simulink model "plataforma"  (R2015a)
settings: Solver=ode45  StartTime=0.0  StopTime=tf  MaxStep=1e-1  RelTol=1e-3
InitFcn:
  | c = clock;
  | seed_offset = c(6);
  | seed_offset = floor(seed_offset);
values from neighbouring files (symbols this model uses):
  Ts = 0.05    [Estimador.m]    (also in Estimador2.m; gerar_realizacao.m; ler_realizacao.m)
settings Model: Creator=marcos  LastModifiedBy=marcos

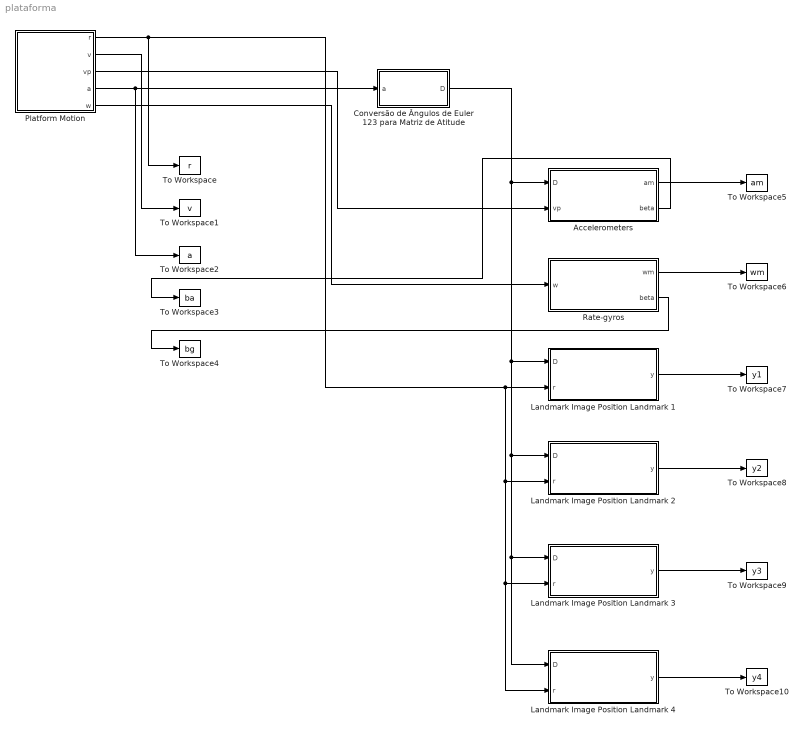
== system plataforma ==
  Accelerometers : Subsystem  mask{beta=zeros(3,1), sigma=0.0039, seed=1+seed_offset}
      mask prompts: beta "Bias (beta)"; sigma "Noise std. dev. (sigma)"
  Conversão de Ângulos de Euler 123 para Matriz de Atitude : MATLAB Function  TreatAsAtomicUnit=on
  Landmark Image Position Landmark 1 : Subsystem  mask{f=1, Dcp=[1 0 0;0 -1 0;0 0 -1], rcp_P=[0 0 0]', sigma=6e-3, p=[0 0 0]', seed=3+seed_offset}
      mask prompts: f "Comprimento focal (f)"; Dcp "Orientação da câmera (Dcp)"; rcp_P "Posição da câmera (rcp)"; sigma "Dev. padrão do ruído (sigma)"; p "Posição da landmark (p)"
  Landmark Image Position Landmark 2 : Subsystem  mask{f=1, Dcp=[1 0 0;0 -1 0;0 0 -1], rcp_P=[0 0 0]', sigma=6e-3, p=[5 5 0]', seed=4+seed_offset}
      mask prompts: f "Comprimento focal (f)"; Dcp "Orientação da câmera (Dcp)"; rcp_P "Posição da câmera (rcp)"; sigma "Dev. padrão do ruído (sigma)"; p "Posição da landmark (p)"
  Landmark Image Position Landmark 3 : Subsystem  mask{f=1, Dcp=[1 0 0;0 -1 0;0 0 -1], rcp_P=[0 0 0]', sigma=6e-3, p=[-5 5 0]', seed=5+seed_offset}
      mask prompts: f "Comprimento focal (f)"; Dcp "Orientação da câmera (Dcp)"; rcp_P "Posição da câmera (rcp)"; sigma "Dev. padrão do ruído (sigma)"; p "Posição da landmark (p)"
  Landmark Image Position Landmark 4 : Subsystem  mask{f=1, Dcp=[1 0 0;0 -1 0;0 0 -1], rcp_P=[0 0 0]', sigma=6e-3, p=[-5 -5 0]', seed=6+seed_offset}
      mask prompts: f "Comprimento focal (f)"; Dcp "Orientação da câmera (Dcp)"; rcp_P "Posição da câmera (rcp)"; sigma "Dev. padrão do ruído (sigma)"; p "Posição da landmark (p)"
  Platform Motion : Subsystem
  Rate-gyros : Subsystem  mask{beta=0.01*ones(3,1), sigma=1e-3, seed=2+0*seed_offset}
      mask prompts: beta "Bias (beta)"; sigma "Noise std. dev. (sigma)"
  To Workspace : ToWorkspace  VariableName=r  SaveFormat=Structure With Time  SampleTime=Ts
  To Workspace1 : ToWorkspace  VariableName=v  SaveFormat=Structure With Time  SampleTime=Ts
  To Workspace10 : ToWorkspace  VariableName=y4  SaveFormat=Structure With Time  SampleTime=Ts
  To Workspace2 : ToWorkspace  VariableName=a  SaveFormat=Structure With Time  SampleTime=Ts
  To Workspace3 : ToWorkspace  VariableName=ba  SaveFormat=Structure With Time  SampleTime=Ts
  To Workspace4 : ToWorkspace  VariableName=bg  SaveFormat=Structure With Time  SampleTime=Ts
  To Workspace5 : ToWorkspace  VariableName=am  SaveFormat=Structure With Time  SampleTime=Ts
  To Workspace6 : ToWorkspace  VariableName=wm  SaveFormat=Structure With Time  SampleTime=Ts
  To Workspace7 : ToWorkspace  VariableName=y1  SaveFormat=Structure With Time  SampleTime=Ts
  To Workspace8 : ToWorkspace  VariableName=y2  SaveFormat=Structure With Time  SampleTime=Ts
  To Workspace9 : ToWorkspace  VariableName=y3  SaveFormat=Structure With Time  SampleTime=Ts
  wires:
  Platform Motion/4(a) -> To Workspace2/1, Conversão de Ângulos de Euler 123 para Matriz de Atitude/1(a)
  Platform Motion/3(vp) -> Accelerometers/2(vp)
  Platform Motion/5(w) -> Rate-gyros/1(w)
  Platform Motion/2(v) -> To Workspace1/1
  Accelerometers/2(beta) -> To Workspace3/1
  Rate-gyros/2(beta) -> To Workspace4/1
  Accelerometers/1(am) -> To Workspace5/1
  Rate-gyros/1(wm) -> To Workspace6/1
  Landmark Image Position Landmark 1/1(y) -> To Workspace7/1
  Landmark Image Position Landmark 2/1(y) -> To Workspace8/1
  Landmark Image Position Landmark 3/1(y) -> To Workspace9/1
  Landmark Image Position Landmark 4/1(y) -> To Workspace10/1
  Platform Motion/1(r) -> To Workspace/1, Landmark Image Position Landmark 4/2(r), Landmark Image Position Landmark 3/2(r), Landmark Image Position Landmark 2/2(r), Landmark Image Position Landmark 1/2(r)
  Conversão de Ângulos de Euler 123 para Matriz de Atitude/1(D) -> Landmark Image Position Landmark 4/1(D), Landmark Image Position Landmark 3/1(D), Landmark Image Position Landmark 2/1(D), Landmark Image Position Landmark 1/1(D), Accelerometers/1(D)

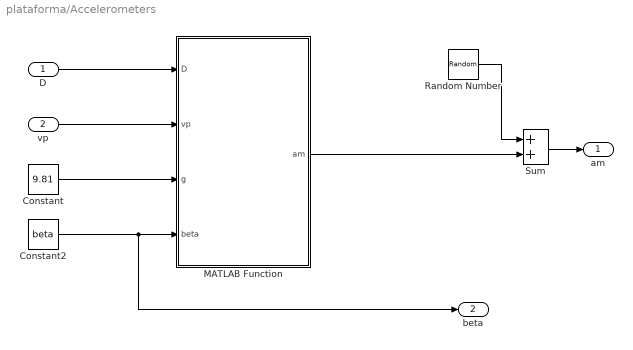
== system plataforma/Accelerometers ==
  D : Inport
  vp : Inport  Port=2
  Constant : Constant  Value=9.81
  Constant2 : Constant  Value=beta
  MATLAB Function : MATLAB Function  TreatAsAtomicUnit=on
  Random Number : RandomNumber  Mean=[0 0 0]'  Variance="[sigma^2  sigma^2  sigma^2]'"  Seed=seed
  Sum : Sum
  am : Outport
  beta : Outport  Port=2
  wires:
  D/1 -> MATLAB Function/1(D)
  vp/1 -> MATLAB Function/2(vp)
  MATLAB Function/1(am) -> Sum/2
  Constant/1 -> MATLAB Function/3(g)
  Constant2/1 -> beta/1, MATLAB Function/4(beta)
  Random Number/1 -> Sum/1
  Sum/1 -> am/1

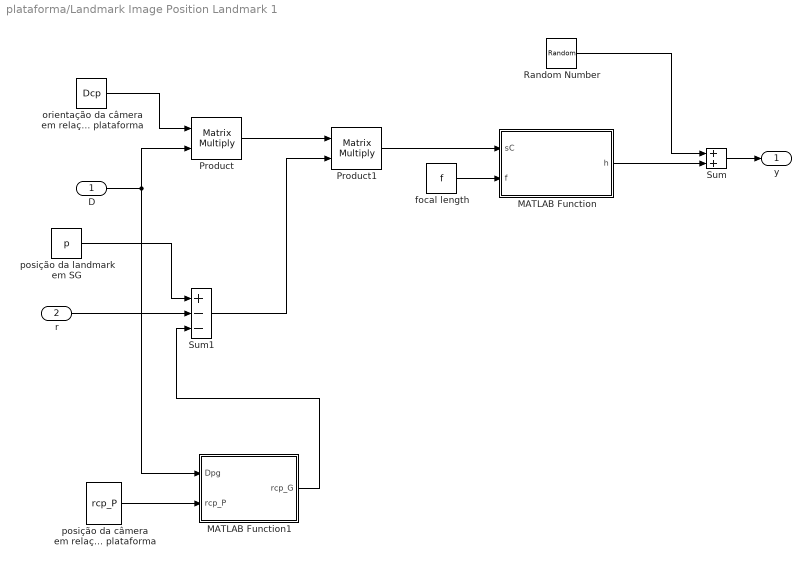
== system plataforma/Landmark Image Position Landmark 1 ==
  D : Inport
  r : Inport  Port=2
  MATLAB Function : MATLAB Function  TreatAsAtomicUnit=on
  MATLAB Function1 : MATLAB Function  TreatAsAtomicUnit=on
  Product : Product  Multiplication=Matrix(*)
  Product1 : Product  Multiplication=Matrix(*)
  Random Number : RandomNumber  Mean=[0 0]'  Variance=[sigma^2 sigma^2]'  Seed=seed
  Sum : Sum
  Sum1 : Sum  Inputs=+--
  focal length : Constant  Value=f
  orientação da câmera em relação à plataforma : Constant  Value=Dcp
  posição da câmera em relação à plataforma : Constant  Value=rcp_P
  posição da landmark em SG : Constant  Value=p
  y : Outport
  wires:
  focal length/1 -> MATLAB Function/2(f)
  MATLAB Function/1(h) -> Sum/2
  Random Number/1 -> Sum/1
  Sum/1 -> y/1
  orientação da câmera em relação à plataforma/1 -> Product/1
  D/1 -> Product/2, MATLAB Function1/1(Dpg)
  Product/1 -> Product1/1
  posição da landmark em SG/1 -> Sum1/1
  r/1 -> Sum1/2
  Sum1/1 -> Product1/2
  Product1/1 -> MATLAB Function/1(sC)
  posição da câmera em relação à plataforma/1 -> MATLAB Function1/2(rcp_P)
  MATLAB Function1/1(rcp_G) -> Sum1/3

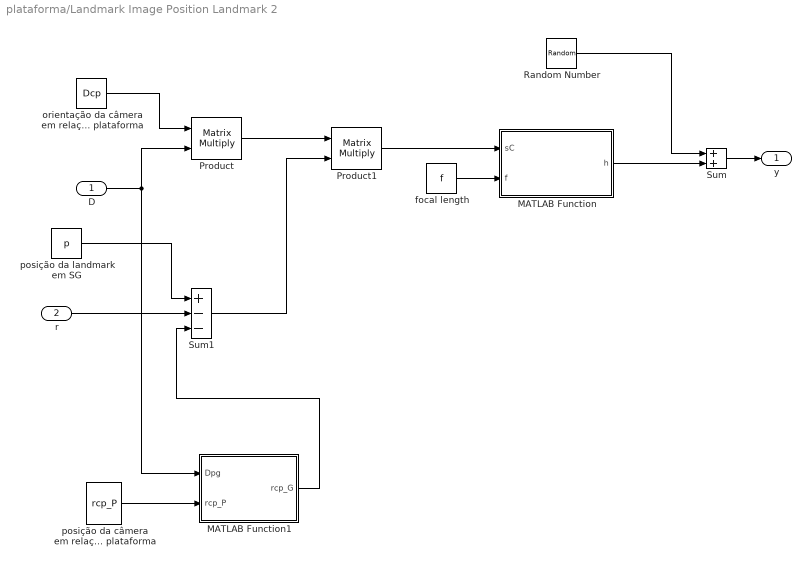
== system plataforma/Landmark Image Position Landmark 2 ==
  D : Inport
  r : Inport  Port=2
  MATLAB Function : MATLAB Function  TreatAsAtomicUnit=on
  MATLAB Function1 : MATLAB Function  TreatAsAtomicUnit=on
  Product : Product  Multiplication=Matrix(*)
  Product1 : Product  Multiplication=Matrix(*)
  Random Number : RandomNumber  Mean=[0 0]'  Variance=[sigma^2 sigma^2]'  Seed=seed
  Sum : Sum
  Sum1 : Sum  Inputs=+--
  focal length : Constant  Value=f
  orientação da câmera em relação à plataforma : Constant  Value=Dcp
  posição da câmera em relação à plataforma : Constant  Value=rcp_P
  posição da landmark em SG : Constant  Value=p
  y : Outport
  wires:
  MATLAB Function1/1(rcp_G) -> Sum1/3
  posição da câmera em relação à plataforma/1 -> MATLAB Function1/2(rcp_P)
  Product1/1 -> MATLAB Function/1(sC)
  Sum1/1 -> Product1/2
  r/1 -> Sum1/2
  posição da landmark em SG/1 -> Sum1/1
  Product/1 -> Product1/1
  D/1 -> MATLAB Function1/1(Dpg), Product/2
  orientação da câmera em relação à plataforma/1 -> Product/1
  Sum/1 -> y/1
  Random Number/1 -> Sum/1
  MATLAB Function/1(h) -> Sum/2
  focal length/1 -> MATLAB Function/2(f)

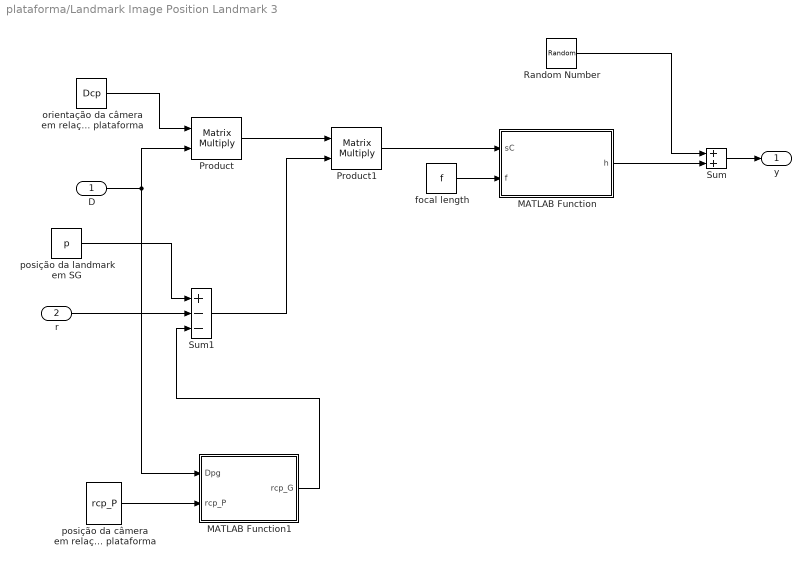
== system plataforma/Landmark Image Position Landmark 3 ==
  D : Inport
  r : Inport  Port=2
  MATLAB Function : MATLAB Function  TreatAsAtomicUnit=on
  MATLAB Function1 : MATLAB Function  TreatAsAtomicUnit=on
  Product : Product  Multiplication=Matrix(*)
  Product1 : Product  Multiplication=Matrix(*)
  Random Number : RandomNumber  Mean=[0 0]'  Variance=[sigma^2 sigma^2]'  Seed=seed
  Sum : Sum
  Sum1 : Sum  Inputs=+--
  focal length : Constant  Value=f
  orientação da câmera em relação à plataforma : Constant  Value=Dcp
  posição da câmera em relação à plataforma : Constant  Value=rcp_P
  posição da landmark em SG : Constant  Value=p
  y : Outport
  wires:
  MATLAB Function1/1(rcp_G) -> Sum1/3
  posição da câmera em relação à plataforma/1 -> MATLAB Function1/2(rcp_P)
  Product1/1 -> MATLAB Function/1(sC)
  Sum1/1 -> Product1/2
  r/1 -> Sum1/2
  posição da landmark em SG/1 -> Sum1/1
  Product/1 -> Product1/1
  D/1 -> MATLAB Function1/1(Dpg), Product/2
  orientação da câmera em relação à plataforma/1 -> Product/1
  Sum/1 -> y/1
  Random Number/1 -> Sum/1
  MATLAB Function/1(h) -> Sum/2
  focal length/1 -> MATLAB Function/2(f)

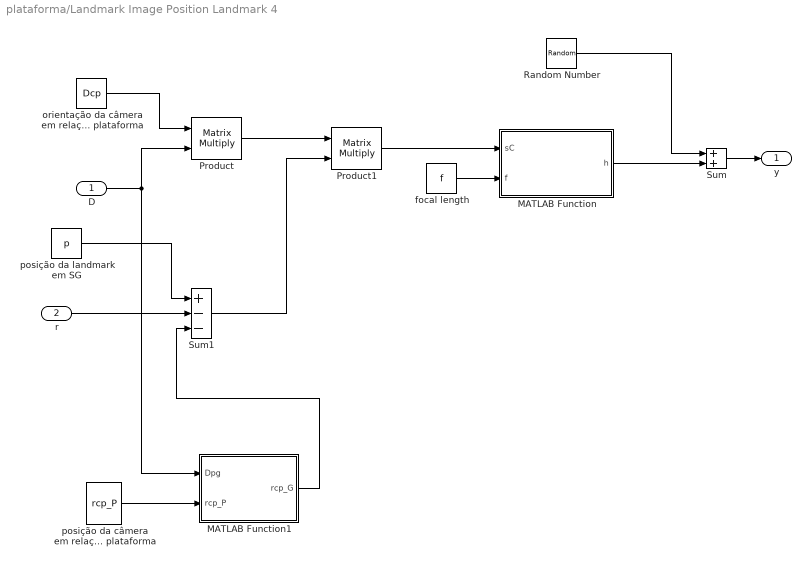
== system plataforma/Landmark Image Position Landmark 4 ==
  D : Inport
  r : Inport  Port=2
  MATLAB Function : MATLAB Function  TreatAsAtomicUnit=on
  MATLAB Function1 : MATLAB Function  TreatAsAtomicUnit=on
  Product : Product  Multiplication=Matrix(*)
  Product1 : Product  Multiplication=Matrix(*)
  Random Number : RandomNumber  Mean=[0 0]'  Variance=[sigma^2 sigma^2]'  Seed=seed
  Sum : Sum
  Sum1 : Sum  Inputs=+--
  focal length : Constant  Value=f
  orientação da câmera em relação à plataforma : Constant  Value=Dcp
  posição da câmera em relação à plataforma : Constant  Value=rcp_P
  posição da landmark em SG : Constant  Value=p
  y : Outport
  wires:
  MATLAB Function1/1(rcp_G) -> Sum1/3
  posição da câmera em relação à plataforma/1 -> MATLAB Function1/2(rcp_P)
  Product1/1 -> MATLAB Function/1(sC)
  Sum1/1 -> Product1/2
  r/1 -> Sum1/2
  posição da landmark em SG/1 -> Sum1/1
  Product/1 -> Product1/1
  D/1 -> MATLAB Function1/1(Dpg), Product/2
  orientação da câmera em relação à plataforma/1 -> Product/1
  Sum/1 -> y/1
  Random Number/1 -> Sum/1
  MATLAB Function/1(h) -> Sum/2
  focal length/1 -> MATLAB Function/2(f)

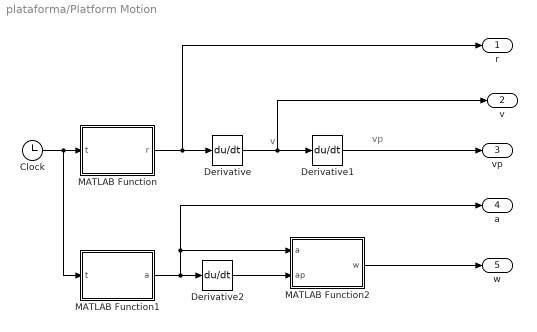
== system plataforma/Platform Motion ==
  note: vp
  note: v
  Clock : Clock
  Derivative : Derivative
  Derivative1 : Derivative
  Derivative2 : Derivative
  MATLAB Function : MATLAB Function  TreatAsAtomicUnit=on
  MATLAB Function1 : MATLAB Function  TreatAsAtomicUnit=on
  MATLAB Function2 : MATLAB Function  TreatAsAtomicUnit=on
  r : Outport
  v : Outport  Port=2
  vp : Outport  Port=3
  a : Outport  Port=4
  w : Outport  Port=5
  wires:
  Clock/1 -> MATLAB Function1/1(t), MATLAB Function/1(t)
  Derivative1/1 -> vp/1
  Derivative2/1 -> MATLAB Function2/2(ap)
  MATLAB Function2/1(w) -> w/1
  MATLAB Function1/1(a) -> a/1, MATLAB Function2/1(a), Derivative2/1
  Derivative/1 -> v/1, Derivative1/1
  MATLAB Function/1(r) -> r/1, Derivative/1

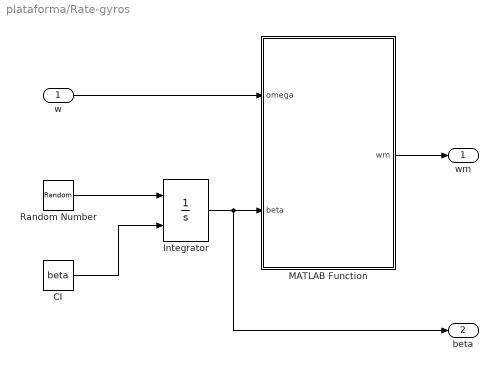
== system plataforma/Rate-gyros ==
  w : Inport
  CI : Constant  Value=beta
  Integrator : Integrator  InitialConditionSource=external
  MATLAB Function : MATLAB Function  TreatAsAtomicUnit=on
  Random Number : RandomNumber  Mean=[0 0 0]'  Variance="[sigma^2  sigma^2  sigma^2]'"  Seed=seed
  wm : Outport
  beta : Outport  Port=2
  wires:
  w/1 -> MATLAB Function/1(omega)
  MATLAB Function/1(wm) -> wm/1
  Integrator/1 -> beta/1, MATLAB Function/2(beta)
  Random Number/1 -> Integrator/1
  CI/1 -> Integrator/2

== matlab function plataforma/Landmark Image Position Landmark 1/MATLAB Function1 ==
  data: Dpg input; rcp_G output; rcp_P input
function rcp_G = fcn(Dpg,rcp_P)
%#codegen

rcp_G = Dpg'*rcp_P;

== matlab function plataforma/Landmark Image Position Landmark 3/MATLAB Function ==
  data: sC input; h output; f input
function h = fcn(sC,f)
%#codegen

h = f/sC(3)*[sC(1);sC(2)];

== matlab function plataforma/Landmark Image Position Landmark 2/MATLAB Function ==
  data: sC input; h output; f input
function h = fcn(sC,f)
%#codegen

h = f/sC(3)*[sC(1);sC(2)];

== matlab function plataforma/Platform Motion/MATLAB Function ==
  data: t input; r output
function r = position(t)
%#codegen

% trajectória de posição, em S_G, em metros

Ax = 5;
Ay = 5;
Az = 1;
h = 20;


r = [Ax*sin(2*pi/20*t);
     Ay*cos(2*pi/20*t);
     Az*sin(2*pi/4*t) + h];

== matlab function plataforma/Platform Motion/MATLAB Function1 ==
  data: t input; a output
function a = attitude(t)
%#codegen

% trajectória de atitude de S_P em relação a S_G, em rad

Afi = pi/18;
Ateta = pi/18;
Apsi = pi/18;

a = [Afi*sin(2*pi/2*t);
     Ateta*cos(2*pi/2*t);
     Apsi*sin(2*pi/8*t)];

== matlab function plataforma/Landmark Image Position Landmark 2/MATLAB Function1 ==
  data: Dpg input; rcp_G output; rcp_P input
function rcp_G = fcn(Dpg,rcp_P)
%#codegen

rcp_G = Dpg'*rcp_P;

== matlab function plataforma/Platform Motion/MATLAB Function2 ==
  data: a input; ap input; w output
function w = angvel(a,ap)
%#codegen

% velocidade angular, em S_P, em rad/s


ca2 = cos(a(2));
ca3 = cos(a(3));
sa2 = sin(a(2));
sa3 = sin(a(3));

Ainv = [ca2*ca3, sa3, 0;
        -ca2*sa3, ca3, 0;
         sa2, 0, 1];
     
w = Ainv*ap;

== matlab function plataforma/Landmark Image Position Landmark 3/MATLAB Function1 ==
  data: Dpg input; rcp_G output; rcp_P input
function rcp_G = fcn(Dpg,rcp_P)
%#codegen

rcp_G = Dpg'*rcp_P;

== matlab function plataforma/Accelerometers/MATLAB Function ==
  data: D input; am output; vp input; g input; beta input
function am = fcn(D,vp,g,beta)
%#codegen

g_G = [0;0;-g];

am = D*(vp - g_G) + beta;

== matlab function plataforma/Rate-gyros/MATLAB Function ==
  data: omega input; wm output; beta input
function wm = fcn(omega,beta)
%#codegen

wm = omega + beta;

== matlab function plataforma/Landmark Image Position Landmark 1/MATLAB Function ==
  data: sC input; h output; f input
function h = fcn(sC,f)
%#codegen

h = f/sC(3)*[sC(1);sC(2)];

== matlab function plataforma/Landmark Image Position Landmark 4/MATLAB Function ==
  data: sC input; h output; f input
function h = fcn(sC,f)
%#codegen

h = f/sC(3)*[sC(1);sC(2)];

== matlab function plataforma/Landmark Image Position Landmark 4/MATLAB Function1 ==
  data: Dpg input; rcp_G output; rcp_P input
function rcp_G = fcn(Dpg,rcp_P)
%#codegen

rcp_G = Dpg'*rcp_P;

== matlab function plataforma/Conversão de Ângulos de Euler 123 para Matriz de Atitude ==
  data: a input; D output
function D  = a1232D(a)

phi = a(1);
theta = a(2);
psi = a(3);

% conversão de ângulos de Euler 123 para matriz de atitude D

D = [cos(psi)*cos(theta), cos(psi)*sin(theta)*sin(phi)+sin(psi)*cos(phi), -cos(psi)*sin(theta)*cos(phi)+sin(psi)*sin(phi);
    -sin(psi)*cos(theta), -sin(psi)*sin(theta)*sin(phi)+cos(psi)*cos(phi), sin(psi)*sin(theta)*cos(phi)+cos(psi)*sin(phi);
    sin(theta) , -cos(theta)*sin(phi), cos(theta)*cos(phi)];
